simulink model "VehicleModel"  (R2016b)
settings: Solver=FixedStepAuto  StartTime=0.0  StopTime=t_EndSimulation  FixedStep=base_dT  MaxStep=0.01  RelTol=1e-3  EnableMultiTasking=on
values from neighbouring files (symbols this model uses):
  b_E2C_inloop = Simulink.Parameter    [VehicleModelInit.m]
  b_Engine_in_loop = Simulink.Parameter    [VehicleModelInit.m]
  b_initialize_distance_t_startsim = Simulink.Parameter    [VehicleModelInit.m]
  b_Ne_in_loop = Simulink.Parameter    [VehicleModelInit.m]
  b_TTB_in_loop = Simulink.Parameter    [VehicleModelInit.m]
  b_use_acc = Simulink.Parameter    [VehicleModelInit.m]
  b_use_acc_hardset = Simulink.Parameter    [VehicleModelInit.m]
  base_dT = Simulink.Parameter    [VehicleModelInit.m]
  c_acc_d_hdw = Simulink.Parameter    [VehicleModelInit.m]
  c_acc_hdw = Simulink.Parameter    [VehicleModelInit.m]
  c_EngFricCoef = PARS.c_EngFricCoef    [VehicleModelInit.m]
  c_EngFricCoefd = PARS.c_EngFricCoefd    [VehicleModelInit.m]
  d_Ne_max = Simulink.Parameter    [VehicleModelInit.m]
  d_Ne_min = Simulink.Parameter    [VehicleModelInit.m]
  Driver_TuneG1 = PARS.Driver_TuneG1    [VehicleModelInit.m]
  Driver_TuneG2 = PARS.Driver_TuneG2    [VehicleModelInit.m]
  Driver_TuneG3 = PARS.Driver_TuneG3    [VehicleModelInit.m]
  Driver_TuneG_aw = PARS.Driver_TuneG_aw    [VehicleModelInit.m]
  E2C_c2_dTB = Simulink.Parameter    [VehicleModelInit.m]
  E2C_c_dTB = Simulink.Parameter    [VehicleModelInit.m]
  E2C_CycleTimespan = Simulink.Parameter    [VehicleModelInit.m]
  E2C_initializeRelDist = Simulink.Parameter    [VehicleModelInit.m]
  E2C_SpeedShape = Simulink.Parameter    [VehicleModelInit.m]
  E2C_Trap_CycleAcceEndAlpha = Simulink.Parameter    [VehicleModelInit.m]
  E2C_Trap_CycleAcceStartAlpha = Simulink.Parameter    [VehicleModelInit.m]
  E2C_Trap_CycleDeceEndAlpha = Simulink.Parameter    [VehicleModelInit.m]
  E2C_Trap_CycleDeceStartAlpha = Simulink.Parameter    [VehicleModelInit.m]
  E2C_V_High_kmh = Simulink.Parameter    [VehicleModelInit.m]
  E2C_V_Low_kmh = Simulink.Parameter    [VehicleModelInit.m]
  E2C_V_max = Simulink.Parameter    [VehicleModelInit.m]
  E2C_V_min = Simulink.Parameter    [VehicleModelInit.m]
  FTP_speed_1sec = [FTP_speed_once.speed;Idle_speed_once;FTP_speed_once.speed;Idle_speed_once;FTP_speed_once.speed]    [VehicleModelInit.m]
  mass = 3123*1.3    (= 4059.9)    [VehicleModelInit.m]
  T_ACC_TuneG1_data = Simulink.Parameter    [VehicleModelInit.m]
  T_ACC_TuneG1_pt = Simulink.Parameter    [VehicleModelInit.m]
  T_ACC_TuneG2_data = Simulink.Parameter    [VehicleModelInit.m]
  T_ACC_TuneG2_pt = Simulink.Parameter    [VehicleModelInit.m]
  t_StartSimulation = Simulink.Parameter    [VehicleModelInit.m]
  T_TB_ego_ini = Simulink.Parameter    [VehicleModelInit.m]
  T_TB_OffSet = Simulink.Parameter    [VehicleModelInit.m]
  tau_EngTorque = Simulink.Parameter    [VehicleModelInit.m]
  tau_Ne = Simulink.Parameter    [VehicleModelInit.m]
  tau_pedal_dem = Simulink.Parameter    [VehicleModelInit.m]
  VESP_MD = x0.VESP    [VehicleModelInit.m]
undefined symbols (not defined in the file or in its folder): Continuous, DiscIntNeverNeededParam, initializeRelDist, p_ego_ini, p_lead_ini, PedalMapMD, r_w, Simulation_dT, spsSampleAndHoldModel, v_lead_ini, x0
libraries: simulink x9, spsEdgeDetectorModel x6, dspsigops x1
(part 1 of 7)
settings Model: Creator=akshart  LastModifiedBy=Hcn
settings DataIOCC: LimitDataPoints=on  SaveFormat=Array  SignalLoggingSaveFormat=ModelDataLogs
settings OptimizationCC: ExpressionDepthLimit=2147483647  InitFltsAndDblsToZero=on  LifeSpan=inf
settings DebuggingCC: UnderspecifiedInitializationDetection=Classic  MergeDetectMultiDrivingBlocksExec=none  SolverPrmCheckMsg=warning  FcnCallInpInsideContextMsg=warning  StateNameClashWarn=warning  SFUnexpectedBacktrackingDiag=warning  SFNoUnconditionalDefaultTransitionDiag=warning  SFExecutionAtInitializationDiag=none
settings HardwareCC: ProdBitPerPointer=32  ProdBitPerSizeT=32  ProdBitPerPtrDiffT=32  ProdLargestAtomicFloat=None  ProdIntDivRoundTo=Undefined  ProdEndianess=Unspecified  ProdWordSize=32  ProdHWDeviceType=32-bit Generic
settings ModelReferenceCC: PropagateSignalLabelsOutOfModel=off
settings GRTTargetCC: TargetLangStandard=C89/C90 (ANSI)  GeneratePreprocessorConditionals=Disable all  CombineOutputUpdateFcns=off  GRTInterface=on
settings ConfigComp: CovMetricSettings=dw  CovHtmlReporting=on  CovSaveCumulativeToWorkspaceVar=on  CovSaveSingleToWorkspaceVar=on  CovExternalEMLEnable=off  CovSFcnEnable=off

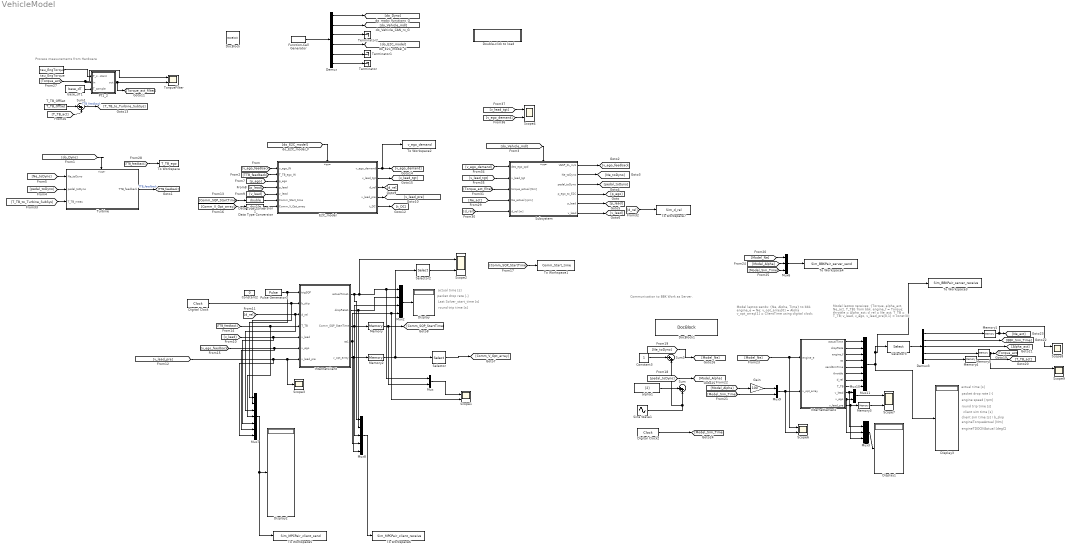
== system VehicleModel ==
  note: Process measurements from Hardware
  note: actual time [s]
  note: packet drop rate [-]
  note: Last Solver_start_time [s]
  note: round trip time [s]
  note: Communication to BBK
      | Work as Server.
  note: Model laptop sends:
      | {Ne, Alpha, Time} to bbk.
      | engine_e = Ne;
      | v_opt_array[0] = Alpha
      | v_opt_array[1] = ClientTime using digital clock;
  note: packet drop rate [-]
  note: actual time [s]
  note: engine speed [rpm]
  note: round trip time [s]
  note: client sim time [s] / b_skip
  note: engineTorqueActual [Nm]
  note: Model laptop receives:
      | {Torque, alpha_act, Ne_act, T_TB} from bbk.
      | engine_f = Torque;
      | throttle = Alpha_act;
      | d_rel = Ne_act;
      | T_TB = T_TB;
      | v_lead, v_ego, v_lead_pre[0,1] = const(0);
  note: engineTDOCINActual [degC]
  note: client sim time [s]
  Constant2 : Constant  Value=0
  Constant3 : Constant
  Data Type Conversion : DataTypeConversion  OutDataTypeStr=double
  Data Type Conversion1 : DataTypeConversion  OutDataTypeStr=double
  Demux : Demux  Outputs=6
  Demux3 : Demux  Outputs=5
  Digital Clock : DigitalClock  SampleTime=base_dT
  Digital Clock2 : DigitalClock  SampleTime=base_dT
  Display{,1..3} (4 alike) : Display
  DocBlock : simulink/Model-Wide Utilities/DocBlock  DocumentType=Text
      content=|
      | Type your documentation here
      |
      | Time                Version Note
      | 101019T1524         Change Ne profile to be slower by changing Driver_Rsl.
      | 101519T2324         Change torque converter torque_ratio in deceleration to make decel Ne fit better.
      | 102219T1600         Integrate solver in Intern_v11 with follower model.
      | 102419T1340         Replace the follower model with 102219T1630 follower model.
      |                     change "off-delay" block to make it run-able in function-call-subsys.
      |                     change multiple continuous solver/integrator to discrete time.
      |                     change multiple delay to discrete time.
      |                     solve "computation loop" problem.
      |                     remove global data store "solver_exec_ctr".
      | 102519T1650         Change the P and I gain for driver_model to be doubled.
      |                     And then changed back, because with the old P and I gains, fuel matches better with data.
      |                     To solve the Ne and speed tracking problem, saturate Ne integrator by 600 and 3400.
      | 102819T1200         Ddd saturation to match idle fuel, only affect fuel consumption number, do not affect driveline.
      |                     Change GearShifting model to have upshift limits: 1600,1800rpm.
      |                     Second bag when vehicle at move (MD.VESP_mph/2.236>=1.5m/s) fuel consumption:
      |                     data fuel at move is -- 764.1621 [g]
      |                     simulink fuel at move is -- 776.5815 [g], +1.63% error.
      | 102819T2340         Change the "follow vehicle1"-->"gain"0.44 place to before acce_filter.
      |                     Previously "filtered_acce" has unit mph/s...
      |                     Change "follow vehicle1"-->"time constant" from 0.5s to 2s.
      |                     data fuel at move is -- 764.5319 [g]
      |                     simulink fuel at move is -- 771.5589 [g], +1.0% error.
      | 102919T1500         -Add substraction for E2C_tiSolverPeriod_C. Because stateflow will add 1 base_dT step.
      |                     Use SendDemand on "E2C_model" subsys to avoid delay introduced by solver_end_time.
      |                     Add function-call subsystem in "E2C_model/solver".
      |                     This way will syncronize with v_ego_array output, and
      |                     update once new optimal v_ego_array is available.
      |                     -"E2C_model/solver/Send  V_demand", add "Matlab Function1" to
      |                     use previous optimal speed as current target speed.
      | 102919T1700         -In previous version, used delayed(v_opt)(1) as previous optimal speed.
      |                     But should be using v_opt(solver_start-delayed(solver_start) ).
      |                     Modified in this version.
      |                     Note: based on solver_start_time to update v_opt_array.
      |                     If solver starts base_dT(s) after solver ends, then correct.
      | 102919T2100         -In previous version, used delayed(v_opt)(1) as previous optimal speed.
      |                     But should be using v_opt(solver_start-delayed(solver_start) ).
      |                     -Use solver_end_time to update v_opt_array.
      | 103119T1400         -Moved leader system out of E2C
      |                     Put leader subsys and Follower subsystem into one function-call system.
      |                     -Compared results from mpcqpsolver and quadprog, final traces are extremely similar. see
      |                     PlatoonModel_Chunan_2016b_102919Txxxx_19_10_31_14_48,PlatoonModel_Chunan_2016b_102919Txxxx_19_10_31_16_22.
      |                     mpcqpsolver is much faster than quadprog.
      | 110519T1100         -in E2C_model, add option for using triditional ACC.
      |                     Add vars b_use_acc,c_acc_hdw.
      |                     changed .m file for setting parameters.
      | 111119T1200         -in E2C_model, add condition for if t_>t_startsimulation.
      |                     only start after 498s.
      |                     -In subsys, change Driver_TuneG1,Driver_TuneG2 to be calibration vars.
      |                     -make V_Opt_Array_modify to be base_dT_delayed(previous V_Opt_Array_modify). Avoid jumps when v_opt updates.
      |                     -PARS.Driver_TuneG1 = 0.015*16;PARS.Driver_TuneG2 = 5;
      |                     with w=0, much smoother optimal speed than before.
      | 111919T1000         -Dyno subsystem change maps for calculating T_TB.
      | 112119T1155         -Add "ToWorkspace" nodes for TTBego, and solver outputs.
      | Client_112619T1415  -Created from PlatoonModel_Chunan_2016b_112119T1155 and InternetClient_112619T1300.
      |                     -Contains the whole vehicle model.
      |                     -Set up memory for CommOut_V_Opt_Array to align change for CommOut_V_Opt_Array and Comm_Start_Time.
      | Solver_112619T1415  -Created.
      |                     -Add semicolon in state flow to avoid printing intermediate variables.
      | C/S_122019T1424     -Add to resolve rtt issue. Not very useful on full model.:
      |                             while (myIns.simTime > timeNow*1)
      |                          {
      |                              QueryPerformanceCounter(&LItNow);
      |                              timeNow = ((double)(LItNow.QuadPart - G.LIstartTime.QuadPart)) / ((double)(G.LIticksPerSecond.QuadPart)) ;
      |                          }
      | %%%%%%%%%%%%%%%%%%%%%%%%%%%%%%%%%%%%%%%%%%%%%%%%%%%%%%%%%%%%%%%%%%%%%%%%%%
      | %                        3-computer setup                                %
      | %%%%%%%%%%%%%%%%%%%%%%%%%%%%%%%%%%%%%%%%%%%%%%%%%%%%%%%%%%%%%%%%%%%%%%%%%%
      | Model_01022020T1343
      |                     -Add Solver block (to bbk).
  DocBlock1 : simulink/Model-Wide Utilities/DocBlock  DocumentType=Text
      content=|
      | 110719T1200         -Finish chart for customized process control
      | 110719T1500         -use Ts=0.1(hardcoded), run server model alone, process control works with EgoFol=1.
      | 110719T1630         -use Ts=base_dT=0.01, run server & client. EgoFol=1.
      | 111119T1200         -Use last_v_opt(solver_start-delayed(solver_start) ) as current v_ego_tgt.
      |                     -Put the modification in Send V_demand subsys.
      |                     -Avoid using another block with detectchange in solver_end_time to trigger this modification.
      |                     -Clean the model and setup communication input/output ports (magenta)
      |                     -Modify Solver_Control so that EgoFol=0 case also works
      | 111119T2200         -Comment out "simulink execution control"
      |                     -If at one step "solver_exec_time>1s", the delay will cumulate
      |                     -need logic control in client to decide whether to skip a trigger.
      | 111219T1300         -Use Client time to set b_termQP.
      |                     -Set E2C_DeltaT=0.3s, save 0.3s for communication
      |                     -Cannot reset if one communication takes long time.
      | Client_112619T1415  -Created from PlatoonModel_Chunan_2016b_112119T1155 and InternetClient_112619T1300.
      |                     -Contains the whole vehicle model.
      |                     -Set up memory for CommOut_V_Opt_Array to align change for CommOut_V_Opt_Array and Comm_Start_Time.
      | Solver_112619T1415  -Created.
      |                     -Add semicolon in state flow to avoid printing intermediate variables.
      | Solver_112719T1142  -Add solver_ctr to workspace
      |                     -Do 10 "dosolver" in 1 step to compensate for base_dT=0.1s. If base_dT=0.01, use 1 dosolver.
      | Solver_112719T2200  -PlatoonModel_Chunan_2016b_112719T2200_solver/Send  V_demand/Triggered Subsystem.
      |                     Change also ceil(current_time-last_start_time).
      | C/S_122019T1424     -Add to resolve rtt issue. Not very useful on full model.:
      |                             while (myIns.simTime > timeNow*1)
      |                          {
      |                              QueryPerformanceCounter(&LItNow);
      |                              timeNow = ((double)(LItNow.QuadPart - G.LIstartTime.QuadPart)) / ((double)(G.LIticksPerSecond.QuadPart)) ;
      |                          }
      | C+S_122019T1618     -Put original solver and client into one system.
      |                     -Now the sent information are place holders to maintain dimension.
      |                     -Finally if this works, the client will be BBK and only sends
      |                     torque, TTB. Solver sends Ne, Alpha.
      | S_122819T1229 (C_122019T1618)
      |                     -Apply changes from Tulga in email "reducing delay further" to 122019T1618.
      |                     -rrt maintains to be 0.02s = base_dT.
      | S_122819T1301 (C_122019T1424)
      |                     -Apply changes from Tulga in email "reducing delay further" to 122019T1424.
      |                     -rrt drops to 0.02s = base_dT.
      |                     -But optimization result is still bad.
      |                     Does not recover optimal results similar to platoonmodel(without interenet),
      |                     like in version S_122819T1229.
      |                     -(!!!)switch Commin_v_lead and v_ego_highfreq at output of InternetServer1 demux.
      | %%%%%%%%%%%%%%%%%%%%%%%%%%%%%%%%%%%%%%%%%%%%%%%%%%%%%%%%%%%%%%%%%%%%%%%%%%
      | %                        3-computer setup                                %
      | %%%%%%%%%%%%%%%%%%%%%%%%%%%%%%%%%%%%%%%%%%%%%%%%%%%%%%%%%%%%%%%%%%%%%%%%%%
  Double-click to load : Subsystem
      settings: OpenFcn=if exist('vesim_init')==2,vesim_init;end;
      mask Help: This block runs/ndes_init.m file in the main directory
      mask Display: disp('Load Input Data')
  E2C_model : Subsystem
  Function-Call Generator : simulink/Ports & Subsystems/Function-Call Generator  sample_time=-1  numberOfIterations=1
  Gain : Gain  Gain=100
  InternetClient : Subsystem  mask(20-sim 4.6 S-Function block){}
      mask help:
      | This block is generated by the 20-sim Matlab Code Generator.
      |
      | * look under the mask to get information on the ports
      | * press Help for more detailed information
      | * the parameters of this block are:
      mask Help:
      | This block is generated by the 20-sim Matlab Code Generator<br>
      | The block parameters are:<br><blockquote></blockquote>
      | Generated at:<br>
      | <blockquote><b>date:  </b>June 14, 2017<br>
      | <b>time:  </b>4:16:43 PM<br></blockquote>
      | From the following 20-sim model:<br>
      | <blockquote><b>submodel:  </b>InternetServer<br>
      | <b>model:  </b>export to Simulink - UM<br>
      | <b>file:  </b>C:\Users\Tulga Ersal\Desktop\For Xueru\export to Simulink - UM.emx<br>
      | <b>experiment:  </b>C:\Users\Tulga Ersal\Desktop\For Xueru\export to Simulink - UM.emx<br></blockquote>
      | Using the following 20-sim license:<br>
      | <blockquote><b>user:  </b>The University of Michigan<br>
      | <b>from:  </b>20-sim 4.6 Student License<br>
      | <b>build: </b>4.6.1.6898<br></blockquote>
  InternetServer2 : Subsystem  mask(20-sim 4.6 S-Function block){}
      mask help:
      | This block is generated by the 20-sim Matlab Code Generator.
      |
      | * look under the mask to get information on the ports
      | * press Help for more detailed information
      | * the parameters of this block are:
      mask Help:
      | This block is generated by the 20-sim Matlab Code Generator<br>
      | The block parameters are:<br><blockquote></blockquote>
      | Generated at:<br>
      | <blockquote><b>date:  </b>June 14, 2017<br>
      | <b>time:  </b>4:16:43 PM<br></blockquote>
      | From the following 20-sim model:<br>
      | <blockquote><b>submodel:  </b>InternetServer<br>
      | <b>model:  </b>export to Simulink - UM<br>
      | <b>file:  </b>C:\Users\Tulga Ersal\Desktop\For Xueru\export to Simulink - UM.emx<br>
      | <b>experiment:  </b>C:\Users\Tulga Ersal\Desktop\For Xueru\export to Simulink - UM.emx<br></blockquote>
      | Using the following 20-sim license:<br>
      | <blockquote><b>user:  </b>The University of Michigan<br>
      | <b>from:  </b>20-sim 4.6 Student License<br>
      | <b>build: </b>4.6.1.6898<br></blockquote>
  Memory : Memory  InheritSampleTime=on  LinearizeAsDelay=on
  Memory1 : Memory  X0=600
  Memory2 : Memory  X0=zeros(40,1)  InheritSampleTime=on  LinearizeAsDelay=on
  Memory3 : Memory  X0=zeros(2,1)  InheritSampleTime=on  LinearizeAsDelay=on
  Memory4 : Memory  X0=200  InheritSampleTime=on  LinearizeAsDelay=on
  Memory5 : Memory  InheritSampleTime=on  LinearizeAsDelay=on
  Mux : Mux  Inputs=2
  Mux10 : Mux  Inputs=2
  Mux11 : Mux  Inputs=8
  Mux2 : Mux
  Mux3 : Mux  Inputs=3
  Mux6 : Mux  Inputs=3
  Mux7 : Mux  Inputs=7
  Mux8 : Mux  Inputs=5
  Mux9 : Mux  Inputs=2
  PT1_2 : Subsystem  mask(PT1_1){}
  Pulse Generator1 : DiscretePulseGenerator  PulseType=Time based  Period=1  PulseWidth=20  SampleTime=base_dT
  Scope{1..2,4,6..9} (7 alike) : Scope  NumInputPorts=2
  Scope3 : Scope
  Selector : Selector  InputPortWidth=40  IndexOptions=Index vector (dialog)  Indices=[1:40]  OutputSizes=1
  Selector2 : Selector  InputPortWidth=40  IndexOptions=Index vector (dialog)  Indices=[1:10]  OutputSizes=1
  Selector3 : Selector  InputPortWidth=8  IndexOptions=Index vector (dialog)  Indices=[3,5,6,7,8]  OutputSizes=1
  Sine Wave1 : Sin  SampleTime=0
  Subsystem : Subsystem
  Sum : Sum  Inputs=|++
  Sum1 : Sum  Inputs=|++
  Sum3 : Sum  Inputs=|++
  T_TB_OffSet : Constant  Value=T_TB_OffSet
  Terminator : Terminator
  Terminator1 : Terminator
  Terminator2 : Terminator
  To Workspace : ToWorkspace  VariableName=T_TB_ego  SaveFormat=Structure With Time  SampleTime=-1
  To Workspace1 : ToWorkspace  VariableName=Comm_Start_time  SaveFormat=Structure With Time  SampleTime=-1
  To Workspace2 : ToWorkspace  VariableName=v_ego_demand  SaveFormat=Structure With Time  SampleTime=-1
  To Workspace3 : ToWorkspace  VariableName=Sim_BBKPair_server_receive  SaveFormat=Structure With Time  SampleTime=-1
  To Workspace4 : ToWorkspace  VariableName=Sim_BBKPair_server_send  SaveFormat=Structure With Time  SampleTime=-1
  To Workspace5 : ToWorkspace  VariableName=Sim_MPCPair_client_send  SaveFormat=Structure With Time  SampleTime=-1
  To Workspace6 : ToWorkspace  VariableName=Sim_MPCPair_client_receive  SaveFormat=Structure With Time  SampleTime=-1
  To Workspace7 : ToWorkspace  VariableName=Sim_d_rel  SaveFormat=Structure With Time  SampleTime=-1
  "TorqueFilter " : Scope  NumInputPorts=2
  Turbine : Subsystem  TreatAsAtomicUnit=on
  alpha1 : Constant  Value=[2]  VectorParams1D=off  SampleTime=base_dT
  base_dT1 : Constant  Value=base_dT
  tau_EngTorque : Constant  Value=tau_EngTorque
  wires:
  [v_ego_feedback] -> E2C_model/1(v_ego_IN)
  [TTB_feedback] -> E2C_model/2(T_TB_ego_IN)
  Function-Call Generator/1 -> Demux/1
  Demux/1 -> [do_Dyno]
  Demux/2 -> [do_Vehicle_mdl]
  Demux/3 -> Terminator2/1
  Demux/4 -> [do_E2C_model]
  Demux/5 -> Terminator1/1
  Demux/6 -> Terminator/1
  [Ne_toDyno] -> Turbine/1(Ne_toDyno)
  [pedal_toDyno] -> Turbine/2(pedal_toDyno)
  [do_E2C_model] -> E2C_model/Trigger
  [do_Dyno] -> Turbine/Trigger
  [do_Vehicle_mdl] -> Subsystem/Trigger
  E2C_model/1(v_ego_demand) -> [v_ego_demand], To Workspace2/1
  Subsystem/1(VESP_FL_m/s) -> [v_ego_feedback]
  Subsystem/2(Ne_toDyno) -> [Ne_toDyno]
  Subsystem/3(pedal_toDyno) -> [pedal_toDyno]
  Subsystem/4(p_ego_to_E2C) -> [p_ego]
  [v_lead_tgt] -> Subsystem/2(v_lead_tgt)
  [p_ego] -> E2C_model/3(p_ego)
  Subsystem/5(p_lead) -> [p_lead]
  [p_lead] -> E2C_model/4(p_lead)
  Subsystem/6(v_lead) -> [v_lead]
  [v_lead] -> E2C_model/5(v_lead)
  [v_ego_feedback] -> Mux7/6, InternetClient/6(v_ego)
  [TTB_feedback] -> Mux7/4, InternetClient/4(T_TB)
  [d_rel] -> Mux7/3, InternetClient/3(d_rel)
  InternetClient/3(Comm_SQP_StartTime) -> Mux8/3, Mux2/3, Memory/1
  Memory/1 -> Mux/2, [Comm_SQP_StartTime]
  InternetClient/5(v_opt_array) -> Mux8/5, Memory2/1
  [v_lead] -> Mux7/5, InternetClient/5(v_lead)
  Pulse Generator1/1 -> Mux7/1, InternetClient/1(trigSQP)
  InternetClient/1(actualTime1) -> Mux8/1, Scope2/1, Mux/1, Mux2/1
  InternetClient/2(dropRate1) -> Mux8/2, Mux2/2
  InternetClient/4(rtt1) -> Scope1/2, Mux2/4, Mux8/4
  Mux2/1 -> Display/1
  E2C_model/3(d_rel) -> [d_rel]
  E2C_model/4(v_lead_pre) -> [v_lead_pre]
  [Comm_SQP_StartTime] -> Data Type Conversion1/1
  [Comm_V_Opt_array] -> Data Type Conversion/1
  Data Type Conversion/1 -> E2C_model/7(Comm_V_Opt_array)
  Data Type Conversion1/1 -> E2C_model/6(Comm_Start_time)
  Memory2/1 -> Selector/1, Selector2/1
  Mux/1 -> Scope1/1
  [Comm_SQP_StartTime] -> To Workspace1/1
  Selector/1 -> [Comm_V_Opt_array]
  Selector2/1 -> Scope2/2
  Digital Clock/1 -> Mux7/2, InternetClient/2(b_skip)
  Mux6/1 -> To Workspace4/1
  Mux7/1 -> Display2/1, To Workspace5/1
  Mux8/1 -> To Workspace6/1
  Demux3/1 -> Memory1/1
  Demux3/2 -> [BBK_Sim_Time]
  Demux3/3 -> [Alpha_act]
  InternetServer2/3(engine_f) -> Mux11/3
  InternetServer2/4(rtt) -> Mux11/4
  InternetServer2/2(dropRate) -> Mux11/2
  InternetServer2/5(sendSimTime) -> Mux11/5
  InternetServer2/1(actualTime) -> Mux11/1
  InternetServer2/6(throttle) -> Mux11/6
  Mux11/1 -> Display3/1, To Workspace3/1, Selector3/1
  InternetServer2/7(d_rel) -> Mux11/7
  InternetServer2/8(T_TB) -> Mux11/8
  InternetServer2/9(v_lead) -> Mux3/1, Mux10/1
  InternetServer2/10(v_ego) -> Mux3/2, Mux10/2
  InternetServer2/11(v_lead_pre) -> Mux3/3, Memory3/1
  alpha1/1 -> Sum/1
  [Model_Ne] -> Scope6/1, InternetServer2/1(engine_e)
  Selector3/1 -> Demux3/1
  Demux3/5 -> Memory4/1
  Memory4/1 -> [T_TB_act]
  Mux9/1 -> Scope6/2, InternetServer2/2(v_opt_array)
  Sine Wave1/1 -> Sum3/2, Sum/2
  Memory3/1 -> Scope7/2
  Digital Clock2/1 -> [Model_Sim_Time]
  [Model_Sim_Time] -> Mux9/2
  [pedal_toDyno] -> [Model_Alpha]
  Constant3/1 -> Sum3/1
  [Ne_toDyno] -> [Model_Ne]
  [Model_Ne] -> Mux6/1
  [Model_Alpha] -> Mux6/2
  [Model_Sim_Time] -> Mux6/3
  Mux10/1 -> Scope7/1
  Mux3/1 -> Display1/1
  E2C_model/5(t_DC) -> [t_DC]
  [Model_Alpha] -> Gain/1
  Gain/1 -> Mux9/1
  [TTB_feedback] -> To Workspace/1
  PT1_2/1(out) -> [Torque_act_filter], "TorqueFilter "/2
  Demux3/4 -> Memory5/1
  Memory1/1 -> Scope8/1, [Ne_act]
  Memory5/1 -> Scope9/1, [Torque_act]
  [Torque_act] -> "TorqueFilter "/1, PT1_2/2(in)
  tau_EngTorque/1 -> PT1_2/1(T_constant)
  base_dT1/1 -> PT1_2/3(T_sample)
  [d_rel] -> To Workspace7/1
  [v_lead_pre] -> Mux7/7, Scope3/1, InternetClient/7(v_lead_pre)
  [Ne_act] -> Subsystem/4(Ne_actual [rpm])
  [T_TB_act] -> Sum1/2
  T_TB_OffSet/1 -> Sum1/1
  Sum1/1 -> [T_TB_to_Turbine_SubSys]  "TTB_feedback"
  [d_rel] -> Subsystem/5(d_rel [m])
  [Torque_act_filter] -> Subsystem/3(torque_actual [Nm])
  Turbine/1(TTB_feedback) -> [TTB_feedback]  "TTB_feedback"
  [T_TB_to_Turbine_SubSys] -> Turbine/3(T_TB_meas)
  [v_ego_demand] -> Subsystem/1(des_ego_spd)
  E2C_model/2(v_lead_tgt) -> [v_lead_tgt]
  [v_lead_tgt] -> Scope4/1
  [v_ego_demand] -> Scope4/2

== system VehicleModel/Double-click to load ==
  note: double_click to load

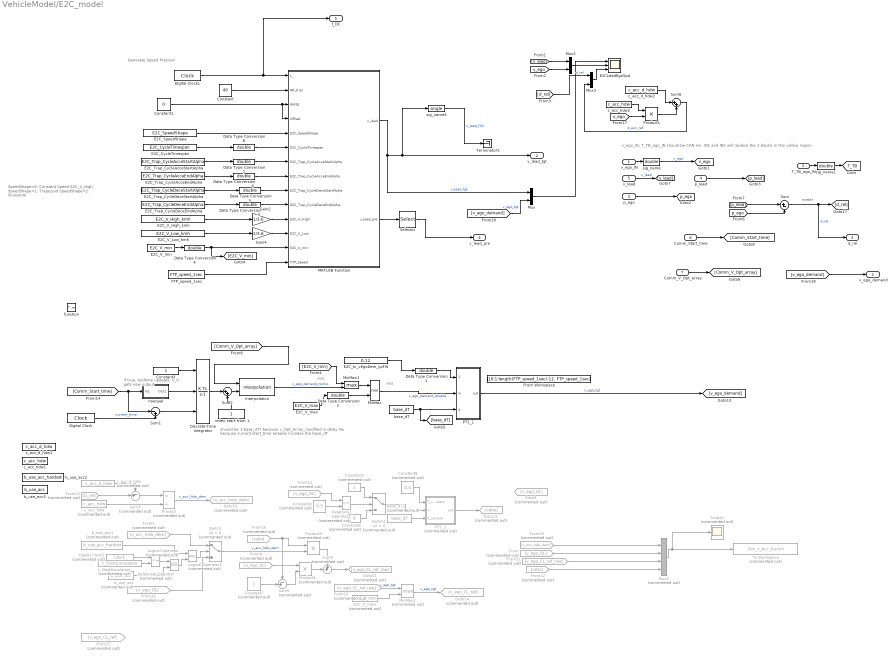
== system VehicleModel/E2C_model ==
  note: should be 1-base_dT? because v_Opt_Array_modified is delay
      | No because current-start_time already includes the base_dT
  note: if true, endtime updates,
      | v_0 gets new output
  note: SpeedShape=0: Constant Speed E2C_V_High
      | SpeedShape=1: Trapezoid
      | SpeedShape=2: Sinusoide
  note: meter
  note: Generate Speed Preview
  note: v_ego_IN, T_TB_ego_IN should be CAN ms. IN1 and IN2 will replace the 2 blocks in this
      | yellow region.
  note: m/s
  note: m/s
  v_ego_IN : Inport
  T_TB_ego_IN : Inport  Port=2
  p_ego : Inport  Port=3
  p_lead : Inport  Port=4
  v_lead : Inport  Port=5
  Comm_Start_time : Inport  Port=6
  Comm_V_Opt_array : Inport  Port=7
  function : TriggerPort  TriggerType=function-call  VariantControl=Variant
  Constant : Constant  Value=40
  Constant1 : Constant  Value=0
  Constant3 : Constant  OutDataTypeStr=double
  Constant4 : Constant  Commented=on  Value=0.5
  Constant5 : Constant  Commented=on
  Constant6 : Constant  Commented=on  Value=0
  Constant7 : Constant  Commented=on
  Constant8 : Constant  Commented=on  Value=0.4
  Data Type Conversion{1..8} (8 alike) : DataTypeConversion  OutDataTypeStr=double
  Digital Clock : DigitalClock  SampleTime=-1
  Digital Clock1 : DigitalClock  SampleTime=-1
  Digital Clock2 : DigitalClock  Commented=on  SampleTime=-1
  Discrete-Time Integrator : DiscreteIntegrator  ExternalReset=rising  InitialConditionSource=external  SampleTime=-1  ICPrevOutput=DiscIntNeverNeededParam  ICPrevScaledInput=DiscIntNeverNeededParam
  E2CLeadEgoSpd : Scope  NumInputPorts=3
  E2C_CycleTimespan : Constant  Value=E2C_CycleTimespan  OutDataTypeStr=single
  E2C_SpeedShape : Constant  Value=E2C_SpeedShape  OutDataTypeStr=uint8
  E2C_Trap_CycleAcceEndAlpha : Constant  Value=E2C_Trap_CycleAcceEndAlpha  OutDataTypeStr=single
  E2C_Trap_CycleAcceStartAlpha : Constant  Value=E2C_Trap_CycleAcceStartAlpha  OutDataTypeStr=single
  E2C_Trap_CycleDeceEndAlpha : Constant  Value=E2C_Trap_CycleDeceEndAlpha  OutDataTypeStr=single
  E2C_Trap_CycleDeceStartAlpha : Constant  Value=E2C_Trap_CycleDeceStartAlpha  OutDataTypeStr=single
  E2C_V_High_kmh : Constant  Value=E2C_V_High_kmh  OutDataTypeStr=single
  E2C_V_Low_kmh : Constant  Value=E2C_V_Low_kmh  OutDataTypeStr=single
  E2C_V_max : Constant  Value=E2C_V_max  OutDataTypeStr=double
  E2C_V_min : Constant  Value=E2C_V_min  OutDataTypeStr=single
  E2C_V_min2 : Constant  Commented=on  Value=E2C_V_min
  E2C_tc_vEgoDem_LpFilt : Constant  Value=0.12  OutDataTypeStr=single
  FTP_speed_1sec : Constant  Value=FTP_speed_1sec
  From{,9,11,16} (4 alike) : From  Commented=on  GotoTag=v_ego_OL
  From Workspace : FromWorkspace  VariableName=[[0:1:length(FTP_speed_1sec)-1]', FTP_speed_1sec]
  From10 : From  Commented=on  GotoTag=v_acc_hdw_dem
  From12 : From  Commented=on  GotoTag=d_rel
  From13 : From  Commented=on  GotoTag=v_ego_CL_ref_raw
  From15 : From  Commented=on  GotoTag=ratio
  From21 : From  Commented=on  GotoTag=v_ego_CL_ref_raw
  From22 : From  Commented=on  GotoTag=ratio
  From25 : From  Commented=on  GotoTag=v_ego_CL_ref
  From5 : From  Commented=on  GotoTag=v_acc_hdw_dem
  Gain2 : Gain  Gain=1/3.6  OutDataTypeStr=double
  Gain4 : Gain  Gain=1/3.6  OutDataTypeStr=double
  Goto10 : Goto  Commented=on  GotoTag=v_acc_hdw_dem
  Goto11 : Goto  Commented=on  GotoTag=v_ego_CL_ref_raw
  Goto12 : Goto  Commented=on  GotoTag=ratio
  Goto14 : Goto  Commented=on  GotoTag=v_ego_CL_ref
  Goto9 : Goto  Commented=on  GotoTag=v_ego_OL
  Interpolation : dspsigops/Interpolation  InterpSource=Input port  InterpPoints=[1.1 4.8 2.67 1.6 3.2]'  InterpMode=Linear  InterpL=3  InterpR=3  InterpAlpha=0.5  InvalidMode=Clip
  Logical Operator : Logic  Commented=on  Operator=OR  AllPortsSameDT=off  OutDataTypeStr=boolean
  Logical Operator1 : Logic  Commented=on  AllPortsSameDT=off  OutDataTypeStr=boolean
  MATLAB Function : MATLAB Function  TreatAsAtomicUnit=on
  MinMax : MinMax  Inputs=2
  MinMax1 : MinMax  Function=max  Inputs=2
  MinMax2 : MinMax  Commented=on  Function=max  Inputs=2
  Mux : Mux  Inputs=2
  Mux1 : Mux  Commented=on
  Mux2 : Mux  Inputs=2
  Mux3 : Mux  Inputs=2
  PT1_1 : Subsystem  mask(PT1_1){}
  PT1_2 : Subsystem  Commented=on  mask(PT1_1){}
  Product : Product  Commented=on  Inputs=*/
  Product1 : Product
  Product3 : Product  Commented=on
  Product4 : Product  Commented=on
  Relational Operator : RelationalOperator  Commented=on  Operator=<=  OutDataTypeStr=boolean  RndMeth=Simplest
  Relational Operator1 : RelationalOperator  Commented=on  OutDataTypeStr=boolean  RndMeth=Simplest
  Scope1 : Scope  Commented=on
  Selector : Selector  InputPortWidth=41  IndexOptions=Index vector (dialog)  Indices=[1:40]  OutputSizes=1
  Sum : Sum  Inputs=|+-
  Sum1 : Sum  Inputs=|-+  OutDataTypeStr=double
  Sum2 : Sum  Inputs=|++
  Sum3 : Sum  Commented=on  Inputs=-+|
  Sum4 : Sum  Commented=on  Inputs=++|
  Sum5 : Sum  Commented=on  Inputs=-+|
  Sum6 : Sum  Inputs=|++
  Switch : Switch  Commented=on  Criteria=u2 > Threshold
  Switch1 : Switch  Commented=on  Criteria=u2 > Threshold
  Terminator5 : Terminator
  To Workspace : ToWorkspace  Commented=on  VariableName=Sim_v_Acc_bunch  SaveFormat=Structure With Time  SampleTime=-1
  b_use_acc : Constant  Commented=on  Value=b_use_acc
  b_use_acc1 : Constant  Commented=on  Value=b_use_acc_hardset
  b_use_acc2 : Constant  Value=b_use_acc_hardset
  b_use_acc3 : Constant  Value=b_use_acc
  base_dT : Constant  Value=base_dT
  base_dT1 : Constant  Commented=on  Value=base_dT
  c_acc_d_hdw : Constant  Commented=on  Value=c_acc_d_hdw
  c_acc_d_hdw1 : Constant  Value=c_acc_d_hdw
  c_acc_d_hdw2 : Constant  Value=c_acc_d_hdw
  c_acc_hdw : Constant  Commented=on  Value=c_acc_hdw
  c_acc_hdw1 : Constant  Value=c_acc_hdw
  c_acc_hdw2 : Constant  Value=c_acc_hdw
  index start from 1 : Constant  OutDataTypeStr=double
  noequal : Subsystem
      mask Display: fprintf('U ~= U/z')
  sig_name : DataTypeConversion  OutDataTypeStr=double
  sig_name1 : DataTypeConversion  OutDataTypeStr=double
  sig_name4 : DataTypeConversion  OutDataTypeStr=single
  t_StartSimulation : Constant  Commented=on  Value=t_StartSimulation
  v_ego_demand : Outport
  v_lead_tgt : Outport  Port=2
  d_rel : Outport  Port=3
  v_lead_pre : Outport  Port=4
  t_DC : Outport  Port=5
  tag scope: T_TB=global, p_ego=global, v_ego=global
  wires:
  [p_ego] -> Sum/2
  [p_lead] -> Sum/1
  T_TB_ego_IN/1 -> sig_name1/1
  sig_name1/1 -> [T_TB]
  v_ego_IN/1 -> sig_name/1
  p_ego/1 -> [p_ego]
  Sum/1 -> d_rel/1, [d_rel]  "d_rel"
  Digital Clock/1 -> Sum1/2  "current_time"
  Constant/1 -> MATLAB Function/2(NP_trial)
  Constant1/1 -> MATLAB Function/4(Offset), MATLAB Function/3(RMSE)
  E2C_SpeedShape/1 -> MATLAB Function/5(E2C_SpeedShape)
  E2C_CycleTimespan/1 -> Data Type Conversion8/1
  E2C_Trap_CycleAcceStartAlpha/1 -> Data Type Conversion7/1
  E2C_Trap_CycleAcceEndAlpha/1 -> Data Type Conversion6/1
  E2C_Trap_CycleDeceStartAlpha/1 -> Data Type Conversion5/1
  E2C_Trap_CycleDeceEndAlpha/1 -> Data Type Conversion3/1
  E2C_V_Low_kmh/1 -> Gain4/1
  E2C_V_min/1 -> Data Type Conversion4/1
  Data Type Conversion4/1 -> [E2C_V_min], MATLAB Function/13(E2C_V_min)
  Gain2/1 -> MATLAB Function/11(E2C_V_High)
  Gain4/1 -> MATLAB Function/12(E2C_V_Low)
  MATLAB Function/2(v_lead_pre) -> Selector/1
  MATLAB Function/1(v_lead) -> Mux/1, v_lead_tgt/1, sig_name4/1  "v_lead_tgt"
  FTP_speed_1sec/1 -> MATLAB Function/14(FTP_Speed)
  E2C_V_High_kmh/1 -> Gain2/1
  Data Type Conversion3/1 -> MATLAB Function/10(E2C_Trap_CycleDeceEndAlpha)
  Data Type Conversion6/1 -> MATLAB Function/8(E2C_Trap_CycleAcceEndAlpha)
  Data Type Conversion5/1 -> MATLAB Function/9(E2C_Trap_CycleDeceStartAlpha)
  Data Type Conversion7/1 -> MATLAB Function/7(E2C_Trap_CycleAcceStartAlpha)
  Data Type Conversion8/1 -> MATLAB Function/6(E2C_CycleTimespan)
  sig_name4/1 -> Terminator5/1  "v_lead_f32"
  [Comm_Start_time] -> Sum1/1, noequal/1(In1)
  Discrete-Time Integrator/1 -> Sum2/1
  index start from 1/1 -> Sum2/2
  Sum2/1 -> Interpolation/2
  Constant3/1 -> Discrete-Time Integrator/1
  [E2C_V_min] -> MinMax1/1
  Interpolation/1 -> MinMax1/2  "v_ego_demand_noclip"
  MinMax1/1 -> MinMax/1
  MinMax/1 -> PT1_1/2(in)  "v_ego_demand_double"
  E2C_tc_vEgoDem_LpFilt/1 -> Data Type Conversion1/1
  base_dT/1 -> PT1_1/3(T_sample), [base_dT]
  E2C_V_max/1 -> Data Type Conversion2/1
  Data Type Conversion2/1 -> MinMax/2
  sig_name/1 -> [v_ego]  "v_ego"
  Data Type Conversion1/1 -> PT1_1/1(T_constant)
  Sum1/1 -> Discrete-Time Integrator/3
  noequal/1(Out1) -> Discrete-Time Integrator/2
  [Comm_V_Opt_array] -> Interpolation/1
  p_lead/1 -> [p_lead]
  v_lead/1 -> [v_lead]  "v_lead"
  Mux/1 -> E2CLeadEgoSpd/1
  Mux2/1 -> E2CLeadEgoSpd/2
  c_acc_hdw/1 -> Product/2
  PT1_1/1(out) -> [v_ego_demand]  "v_ego_tgt"
  Digital Clock1/1 -> t_DC/1, MATLAB Function/1(t_)
  [v_lead] -> Mux2/1
  [v_ego] -> Mux2/2
  Selector/1 -> v_lead_pre/1
  Comm_V_Opt_array/1 -> [Comm_V_Opt_array]
  Comm_Start_time/1 -> [Comm_Start_time]
  E2C_V_min2/1 -> MinMax2/2
  Sum3/1 -> Product/1
  From13/1 -> MinMax2/1  "v_ego_tgt"
  t_StartSimulation/1 -> Relational Operator/2
  Digital Clock2/1 -> Relational Operator/1
  Relational Operator/1 -> Logical Operator/1
  b_use_acc/1 -> Logical Operator/2
  Logical Operator/1 -> Logical Operator1/2
  From12/1 -> Sum3/2
  From16/1 -> Switch/3
  Product/1 -> Goto10/1  "v_acc_hdw_dem"
  Product3/1 -> Sum4/1
  Product4/1 -> Sum4/2
  From/1 -> Mux1/2
  From10/1 -> Mux1/1
  From11/1 -> Relational Operator1/1
  Sum4/1 -> Goto11/1
  Relational Operator1/1 -> Switch1/2
  Constant4/1 -> Relational Operator1/2
  base_dT1/1 -> PT1_2/3(T_sample)
  Constant5/1 -> Switch1/1
  Constant6/1 -> Switch1/3
  Switch1/1 -> PT1_2/2(in)
  PT1_2/1(out) -> Goto12/1
  From9/1 -> Product4/1
  Sum5/1 -> Product4/2
  Constant7/1 -> Sum5/2
  Constant8/1 -> PT1_2/1(T_constant)
  From15/1 -> Sum5/1, Product3/1
  c_acc_d_hdw/1 -> Sum3/1
  Switch/1 -> Product3/2  "v_acc_hdw_dem"
  From5/1 -> Switch/1
  [v_ego_demand] -> Mux/2  "v_ego_tgt"
  Mux1/1 -> Scope1/1, To Workspace/1
  From21/1 -> Mux1/3
  Logical Operator1/1 -> Switch/2
  b_use_acc1/1 -> Logical Operator1/1
  From22/1 -> Mux1/4
  MinMax2/1 -> Goto14/1  "v_ego_tgt"
  [v_ego_demand] -> v_ego_demand/1
  c_acc_hdw2/1 -> Product1/1
  [v_ego] -> Product1/2
  Product1/1 -> Sum6/2
  c_acc_d_hdw2/1 -> Sum6/1
  [d_rel] -> Mux3/1  "d_rel"
  Mux3/1 -> E2CLeadEgoSpd/3
  Sum6/1 -> Mux3/2  "d_acc_ref"

== system VehicleModel/InternetClient ==
  trigSQP : Inport
  b_skip : Inport  Port=2
  d_rel : Inport  Port=3
  T_TB : Inport  Port=4
  v_lead : Inport  Port=5
  v_ego : Inport  Port=6
  v_lead_pre : Inport  Port=7
  Demux1 : Demux  Outputs=[1 1 1 1 40 ]
  Mux1 : Mux  Inputs=[1 1 1 1 1 1 40 ]
  S-Function1 : S-Function  FunctionName=InternetClient  SFunctionDeploymentMode=off  EnableBusSupport=off
  actualTime1 : Outport
  dropRate1 : Outport  Port=2
  Comm_SQP_StartTime : Outport  Port=3
  rtt1 : Outport  Port=4
  v_opt_array : Outport  Port=5
  wires:
  Demux1/1 -> actualTime1/1
  Demux1/2 -> dropRate1/1
  Demux1/3 -> Comm_SQP_StartTime/1
  Demux1/4 -> rtt1/1
  S-Function1/1 -> Demux1/1
  trigSQP/1 -> Mux1/1
  b_skip/1 -> Mux1/2
  Mux1/1 -> S-Function1/1
  T_TB/1 -> Mux1/4
  d_rel/1 -> Mux1/3
  v_lead/1 -> Mux1/5
  v_ego/1 -> Mux1/6
  v_lead_pre/1 -> Mux1/7
  Demux1/5 -> v_opt_array/1

== system VehicleModel/InternetServer2 ==
  engine_e : Inport
  v_opt_array : Inport  Port=2
  Demux : Demux  Outputs=[1 1 1 1 1 1 1 1 1 1 2]
  Mux : Mux  Inputs=[1 2 ]
  S-Function : S-Function  FunctionName=InternetServer  SFunctionDeploymentMode=off  EnableBusSupport=off
  actualTime : Outport
  dropRate : Outport  Port=2
  engine_f : Outport  Port=3
  rtt : Outport  Port=4
  sendSimTime : Outport  Port=5
  throttle : Outport  Port=6
  d_rel : Outport  Port=7
  T_TB : Outport  Port=8
  v_lead : Outport  Port=9
  v_ego : Outport  Port=10
  v_lead_pre : Outport  Port=11
  wires:
  engine_e/1 -> Mux/1
  Demux/1 -> actualTime/1
  Demux/2 -> dropRate/1
  Demux/3 -> engine_f/1
  Demux/4 -> rtt/1
  Demux/5 -> sendSimTime/1
  Demux/6 -> throttle/1
  Mux/1 -> S-Function/1
  S-Function/1 -> Demux/1
  Demux/7 -> d_rel/1
  Demux/8 -> T_TB/1
  Demux/9 -> v_lead/1
  Demux/10 -> v_ego/1
  Demux/11 -> v_lead_pre/1
  v_opt_array/1 -> Mux/2

== system VehicleModel/PT1_2 ==
  T_constant : Inport
  in : Inport  Port=2
  T_sample : Inport  Port=3
  map_error_1 : Sum  Inputs=+-  SaturateOnIntegerOverflow=on  InputSameDT=on  OutDataTypeStr=Inherit: Same as first input
  map_error_2 : Sum  Inputs=2  SaturateOnIntegerOverflow=on  InputSameDT=on  OutDataTypeStr=Inherit: Same as first input
  product_1 : Product  Inputs=*/  SaturateOnIntegerOverflow=on  InputSameDT=on  OutDataTypeStr=Inherit: Same as first input
  product_2 : Product  Inputs=**  SaturateOnIntegerOverflow=on  InputSameDT=on  OutDataTypeStr=Inherit: Same as first input
  saturation_1 : Saturate  UpperLimit=1  LowerLimit=0
  unit_delay_1 : UnitDelay  SampleTime=-1
  out : Outport
  wires:
  T_constant/1 -> product_1/2
  T_sample/1 -> product_1/1
  in/1 -> map_error_1/1
  map_error_1/1 -> product_2/2
  product_1/1 -> saturation_1/1
  saturation_1/1 -> product_2/1
  unit_delay_1/1 -> map_error_1/2, map_error_2/2
  map_error_2/1 -> out/1, unit_delay_1/1
  product_2/1 -> map_error_2/1

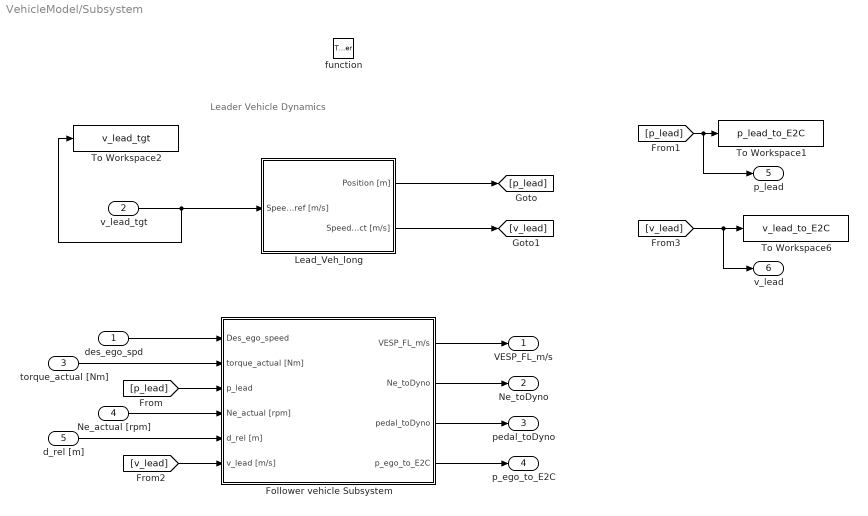
== system VehicleModel/Subsystem ==
  note: Leader Vehicle Dynamics
  des_ego_spd : Inport
  v_lead_tgt : Inport  Port=2
  torque_actual [Nm] : Inport  Port=3
  Ne_actual [rpm] : Inport  Port=4
  d_rel [m] : Inport  Port=5
  function : TriggerPort  TriggerType=function-call  VariantControl=Variant
  Follower vehicle Subsystem : Subsystem  TreatAsAtomicUnit=on
  Lead_Veh_long : Subsystem
  To Workspace1 : ToWorkspace  VariableName=p_lead_to_E2C  SaveFormat=Structure With Time  SampleTime=-1
  To Workspace2 : ToWorkspace  VariableName=v_lead_tgt  SaveFormat=Structure With Time  SampleTime=-1
  To Workspace6 : ToWorkspace  VariableName=v_lead_to_E2C  SaveFormat=Structure With Time  SampleTime=-1
  VESP_FL_m/s : Outport
  Ne_toDyno : Outport  Port=2
  pedal_toDyno : Outport  Port=3
  p_ego_to_E2C : Outport  Port=4
  p_lead : Outport  Port=5
  v_lead : Outport  Port=6
  wires:
  Follower vehicle Subsystem/1(VESP_FL_m/s) -> VESP_FL_m/s/1
  Follower vehicle Subsystem/3(pedal_toDyno) -> pedal_toDyno/1
  Follower vehicle Subsystem/2(Ne_toDyno) -> Ne_toDyno/1
  Lead_Veh_long/1(Position [m]) -> [p_lead]
  v_lead_tgt/1 -> To Workspace2/1, Lead_Veh_long/1(Speed_ref [m/s])
  Follower vehicle Subsystem/4(p_ego_to_E2C) -> p_ego_to_E2C/1
  Lead_Veh_long/2(Speed_act [m/s]) -> [v_lead]
  des_ego_spd/1 -> Follower vehicle Subsystem/1(Des_ego_speed)
  torque_actual [Nm]/1 -> Follower vehicle Subsystem/2(torque_actual [Nm])
  Ne_actual [rpm]/1 -> Follower vehicle Subsystem/4(Ne_actual [rpm])
  d_rel [m]/1 -> Follower vehicle Subsystem/5(d_rel [m])
  [p_lead] -> Follower vehicle Subsystem/3(p_lead)
  [v_lead] -> Follower vehicle Subsystem/6(v_lead [m/s])
  [p_lead] -> p_lead/1, To Workspace1/1
  [v_lead] -> To Workspace6/1, v_lead/1

== system VehicleModel/Turbine ==
  note: Should not use this one for careful simulation tests.
      | This is only needed to setup the code at the first place.
  Ne_toDyno : Inport
  pedal_toDyno : Inport  Port=2
  T_TB_meas : Inport  Port=3
  function : TriggerPort  TriggerType=function-call  VariantControl=Variant
  Constant : Constant  Commented=on  Value=base_dT
  Memory : Memory  Commented=on
  Product : Product  Commented=on  Inputs=/*
  Sum : Sum  Commented=on  Inputs=|-+
  Switch : Switch  Criteria=u2 > Threshold
  TTB : Scope  NumInputPorts=3
  To Workspace8 : ToWorkspace  VariableName=T_TB_ego_Sim  SaveFormat=Structure With Time  SampleTime=-1
  Turbine Thermal : Subsystem  Commented=on
  Turbine Thermal1 : Subsystem
  b_TTB_in_loop : Constant  Value=b_TTB_in_loop  SampleTime=-1
  TTB_feedback : Outport  InitialOutput=200
  wires:
  Turbine Thermal/1(T_TB_ego) -> Turbine Thermal/3(T_TB_ego1)
  Product/1 -> Turbine Thermal/2(a_ego)
  pedal_toDyno/1 -> Turbine Thermal1/2(pedal_ego)
  Ne_toDyno/1 -> Turbine Thermal1/1(Ne_ego)
  Memory/1 -> Sum/1
  Sum/1 -> Product/2
  Constant/1 -> Product/1
  b_TTB_in_loop/1 -> Switch/2
  Turbine Thermal1/1(T_TB_ego) -> TTB/2, Switch/3, To Workspace8/1, Turbine Thermal1/3(T_TB_ego1)  "TTB_sim"
  T_TB_meas/1 -> TTB/1, Switch/1
  Switch/1 -> TTB/3, TTB_feedback/1

== system VehicleModel/E2C_model/PT1_1 ==
  T_constant : Inport
  in : Inport  Port=2
  T_sample : Inport  Port=3
  map_error_1 : Sum  Inputs=+-  SaturateOnIntegerOverflow=on  InputSameDT=on  OutDataTypeStr=Inherit: Same as first input
  map_error_2 : Sum  Inputs=2  SaturateOnIntegerOverflow=on  InputSameDT=on  OutDataTypeStr=Inherit: Same as first input
  product_1 : Product  Inputs=*/  SaturateOnIntegerOverflow=on  InputSameDT=on  OutDataTypeStr=Inherit: Same as first input
  product_2 : Product  Inputs=**  SaturateOnIntegerOverflow=on  InputSameDT=on  OutDataTypeStr=Inherit: Same as first input
  saturation_1 : Saturate  UpperLimit=1  LowerLimit=0
  unit_delay_1 : UnitDelay  SampleTime=-1
  out : Outport
  wires:
  T_constant/1 -> product_1/2
  T_sample/1 -> product_1/1
  in/1 -> map_error_1/1
  map_error_1/1 -> product_2/2
  product_1/1 -> saturation_1/1
  saturation_1/1 -> product_2/1
  unit_delay_1/1 -> map_error_1/2, map_error_2/2
  map_error_2/1 -> out/1, unit_delay_1/1
  product_2/1 -> map_error_2/1

== system VehicleModel/E2C_model/PT1_2 ==
  T_constant : Inport
  in : Inport  Port=2
  T_sample : Inport  Port=3
  map_error_1 : Sum  Inputs=+-  SaturateOnIntegerOverflow=on  InputSameDT=on  OutDataTypeStr=Inherit: Same as first input
  map_error_2 : Sum  Inputs=2  SaturateOnIntegerOverflow=on  InputSameDT=on  OutDataTypeStr=Inherit: Same as first input
  product_1 : Product  Inputs=*/  SaturateOnIntegerOverflow=on  InputSameDT=on  OutDataTypeStr=Inherit: Same as first input
  product_2 : Product  Inputs=**  SaturateOnIntegerOverflow=on  InputSameDT=on  OutDataTypeStr=Inherit: Same as first input
  saturation_1 : Saturate  UpperLimit=1  LowerLimit=0
  unit_delay_1 : UnitDelay  SampleTime=-1
  out : Outport
  wires:
  T_constant/1 -> product_1/2
  T_sample/1 -> product_1/1
  in/1 -> map_error_1/1
  map_error_1/1 -> product_2/2
  product_1/1 -> saturation_1/1
  saturation_1/1 -> product_2/1
  unit_delay_1/1 -> map_error_1/2, map_error_2/2
  map_error_2/1 -> out/1, unit_delay_1/1
  product_2/1 -> map_error_2/1

== system VehicleModel/E2C_model/noequal ==
  In1 : Inport
  Relational Operator : RelationalOperator  Operator=~=  OutDataTypeStr=boolean  RndMeth=Simplest
  Unit Delay : UnitDelay  SampleTime=-1
  Out1 : Outport
  wires:
  Relational Operator/1 -> Out1/1
  Unit Delay/1 -> Relational Operator/2
  In1/1 -> Unit Delay/1, Relational Operator/1

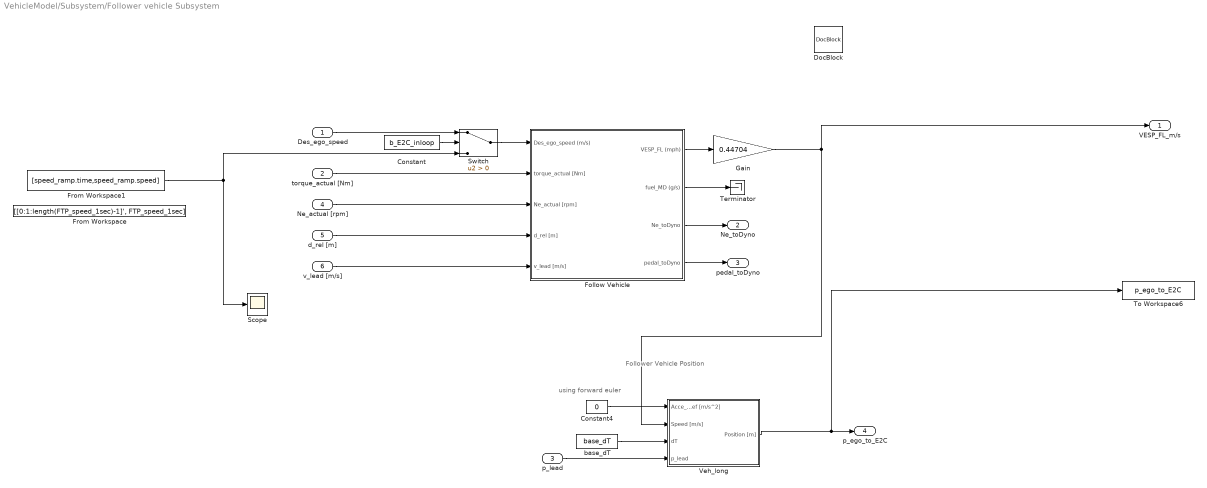
== system VehicleModel/Subsystem/Follower vehicle Subsystem ==
  note: using forward euler
  note: Follower Vehicle Position
  Des_ego_speed : Inport
  torque_actual [Nm] : Inport  Port=2
  p_lead : Inport  Port=3
  Ne_actual [rpm] : Inport  Port=4
  d_rel [m] : Inport  Port=5
  v_lead [m/s] : Inport  Port=6
  Constant : Constant  Value=b_E2C_inloop
  Constant4 : Constant  Value=0
  DocBlock : simulink/Model-Wide Utilities/DocBlock  DocumentType=Text
      content=|
      | Type your documentation here
      |
      | Time
      | 101019T1524         Change Ne profile to be slower by changing Driver_Rsl.
      | 101519T2324         Change torque converter torque_ratio in deceleration to make decel Ne fit better.
      | 102219T1630         Update Gear shift map.
      |                     Use the static Gear shift map depending on (VehV_v,VehV_a)
      |                     Force upshift if engine speed is already >2200 rpm.
      |                     Use filtered V to calculate VehV_a, not the MPC output a_demand.
      | 102519T1650         Change the P and I gain for driver_model to be doubled.
      |                     And then changed back, because with the old P and I gains, fuel matches better with data.
      |                     To solve the Ne and speed tracking problem, saturate Ne integrator by 600 and 3400.
      | 102819T1200         Ddd saturation to match idle fuel, only affect fuel consumption number, do not affect driveline.
      |                     Change GearShifting model to have upshift limits: 1600,1800rpm.
      |                     Second bag when vehicle at move (MD.VESP_mph/2.236>=1.5m/s) fuel consumption:
      |                     data fuel at move is -- 764.1621 [g]
      |                     simulink fuel at move is -- 776.5815 [g], +1.63% error.
      | 102819T2340         Change the "follow vehicle1"-->"gain"0.44 place to before acce_filter.
      |                     Previously "filtered_acce" has unit mph/s...
      |                     Change "follow vehicle1"-->"time constant" from 0.5s to 2s.
      |                     data fuel at move is -- 764.5319 [g]
      |                     simulink fuel at move is -- 771.5589 [g], +1.0% error.
  Follow Vehicle : Subsystem
  From Workspace : FromWorkspace  VariableName=[[0:1:length(FTP_speed_1sec)-1]', FTP_speed_1sec]
  From Workspace1 : FromWorkspace  VariableName=[speed_ramp.time,speed_ramp.speed]
  Gain : Gain  Gain=0.44704
  Scope : Scope
  Switch : Switch  Criteria=u2 > Threshold
  Terminator : Terminator
  To Workspace6 : ToWorkspace  VariableName=p_ego_to_E2C  SaveFormat=Structure With Time  SampleTime=-1
  "Veh_long " : Subsystem
  base_dT : Constant  Value=base_dT
  VESP_FL_m/s : Outport
  Ne_toDyno : Outport  Port=2
  pedal_toDyno : Outport  Port=3
  p_ego_to_E2C : Outport  Port=4
  wires:
  Follow Vehicle/1(VESP_FL (mph)) -> Gain/1
  Follow Vehicle/3(Ne_toDyno) -> Ne_toDyno/1
  Follow Vehicle/4(pedal_toDyno) -> pedal_toDyno/1
  Switch/1 -> Follow Vehicle/1(Des_ego_speed (m/s))
  Des_ego_speed/1 -> Switch/1
  From Workspace1/1 -> Switch/3, Scope/1
  Constant/1 -> Switch/2
  base_dT/1 -> "Veh_long "/3(dT)
  "Veh_long "/1(Position [m]) -> To Workspace6/1, p_ego_to_E2C/1
  Constant4/1 -> "Veh_long "/1(Acce_ref [m/s^2])
  Gain/1 -> VESP_FL_m/s/1, "Veh_long "/2(Speed [m/s])
  torque_actual [Nm]/1 -> Follow Vehicle/2(torque_actual [Nm])
  p_lead/1 -> "Veh_long "/4(p_lead)
  Follow Vehicle/2(fuel_MD (g/s)) -> Terminator/1
  Ne_actual [rpm]/1 -> Follow Vehicle/3(Ne_actual [rpm])
  d_rel [m]/1 -> Follow Vehicle/4(d_rel [m])
  v_lead [m/s]/1 -> Follow Vehicle/5(v_lead [m/s])

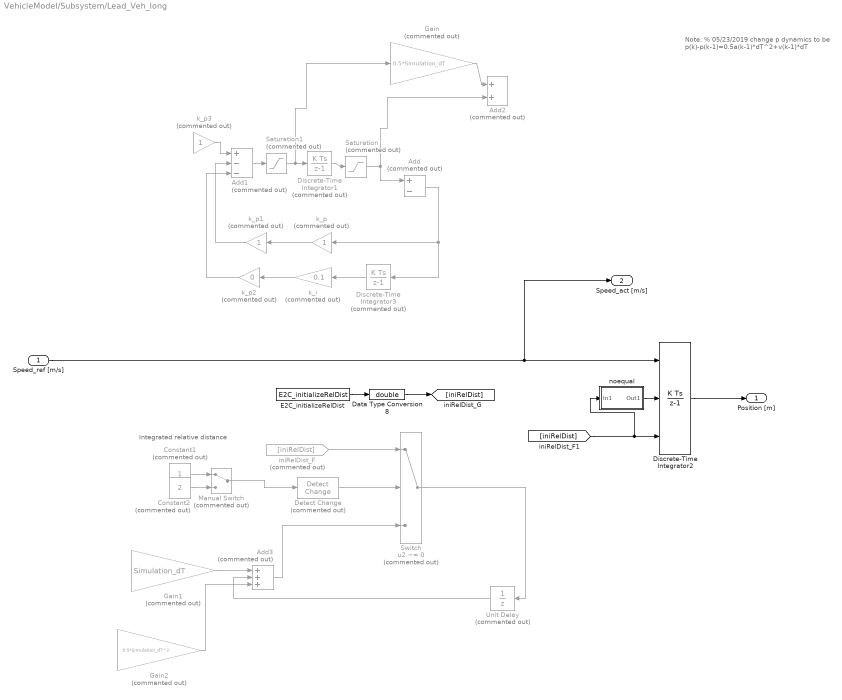
== system VehicleModel/Subsystem/Lead_Veh_long ==
  note: Note:
      | % 05/23/2019
      | change p dynamics to be p(k)-p(k-1)=0.5a(k-1)*dT^2+v(k-1)*dT
  note: Integrated relative distance
  Speed_ref [m/s] : Inport
  Add : Sum  Commented=on  Inputs=+-
  Add1 : Sum  Commented=on  Inputs=+--
  Add2 : Sum  Commented=on
  Add3 : Sum  Commented=on  Inputs=+++
  Constant1 : Constant  Commented=on
  Constant2 : Constant  Commented=on  Value=2
  Data Type Conversion8 : DataTypeConversion  OutDataTypeStr=double
  Detect Change : simulink/Logic and Bit Operations/Detect Change  Commented=on  vinit=0  OutDataTypeStr=boolean
  Discrete-Time Integrator1 : DiscreteIntegrator  Commented=on  InitialCondition=v_lead_ini  InitialConditionSetting=State (most efficient)  SampleTime=-1  ICPrevOutput=DiscIntNeverNeededParam  ICPrevScaledInput=DiscIntNeverNeededParam
  Discrete-Time Integrator2 : DiscreteIntegrator  ExternalReset=rising  InitialConditionSource=external  InitialCondition=p_lead_ini  SampleTime=-1  ICPrevOutput=DiscIntNeverNeededParam  ICPrevScaledInput=DiscIntNeverNeededParam
  Discrete-Time Integrator3 : DiscreteIntegrator  Commented=on  InitialConditionSetting=State (most efficient)  SampleTime=-1  ICPrevOutput=DiscIntNeverNeededParam  ICPrevScaledInput=DiscIntNeverNeededParam
  E2C_initializeRelDist : Constant  Value=E2C_initializeRelDist  OutDataTypeStr=double
  Gain : Gain  Commented=on  Gain=0.5*Simulation_dT
  Gain1 : Gain  Commented=on  Gain=Simulation_dT
  Gain2 : Gain  Commented=on  Gain=0.5*Simulation_dT^2
  Manual Switch : ManualSwitch  Commented=on
  Saturation : Saturate  Commented=on  UpperLimit=30  LowerLimit=0
  Saturation1 : Saturate  Commented=on  UpperLimit=6  LowerLimit=-6
  Switch : Switch  Commented=on  Criteria=u2 ~= 0
  Unit Delay : UnitDelay  Commented=on  SampleTime=-1
  iniRelDist_F : From  Commented=on  GotoTag=iniRelDist
  k_i : Gain  Commented=on  Gain=0.1
  k_p : Gain  Commented=on
  k_p1 : Gain  Commented=on
  k_p2 : Gain  Commented=on  Gain=0
  k_p3 : Gain  Commented=on
  noequal : Subsystem
      mask Display: fprintf('U ~= U/z')
  Position [m] : Outport
  Speed_act [m/s] : Outport  Port=2
  wires:
  Switch/1 -> Unit Delay/1
  Add/1 -> Discrete-Time Integrator3/1, k_p/1
  Discrete-Time Integrator3/1 -> k_i/1
  k_i/1 -> k_p2/1
  k_p/1 -> k_p1/1
  k_p1/1 -> Add1/2
  k_p2/1 -> Add1/3
  Add1/1 -> Saturation1/1
  Discrete-Time Integrator1/1 -> Saturation/1
  k_p3/1 -> Add1/1
  Saturation/1 -> Add2/2, Add/1
  Gain/1 -> Add2/1
  Speed_ref [m/s]/1 -> Speed_act [m/s]/1, Discrete-Time Integrator2/1
  Saturation1/1 -> Discrete-Time Integrator1/1, Gain/1
  iniRelDist_F/1 -> Switch/1
  Detect Change/1 -> Switch/2
  Add3/1 -> Switch/3
  Unit Delay/1 -> Add3/2
  Gain1/1 -> Add3/1
  Gain2/1 -> Add3/3
  Constant1/1 -> Manual Switch/1
  Constant2/1 -> Manual Switch/2
  Manual Switch/1 -> Detect Change/1
  Discrete-Time Integrator2/1 -> Position [m]/1
  [iniRelDist] -> noequal/1(In1), Discrete-Time Integrator2/3
  noequal/1(Out1) -> Discrete-Time Integrator2/2
  E2C_initializeRelDist/1 -> Data Type Conversion8/1
  Data Type Conversion8/1 -> [iniRelDist]

== system VehicleModel/Turbine/Turbine Thermal ==
  v_ego : Inport
  a_ego : Inport  Port=2
  T_TB_ego1 : Inport  Port=3
  Add : Sum  Inputs=+-
  Constant : Constant  Value=T_TB_ego_ini
  Data Type Conversion1 : DataTypeConversion  OutDataTypeStr=double
  Data Type Conversion9 : DataTypeConversion  OutDataTypeStr=double
  Discrete-Time Integrator : DiscreteIntegrator  InitialConditionSource=external  InitialCondition=T_TB_ego_ini  SampleTime=-1  ICPrevOutput=DiscIntNeverNeededParam  ICPrevScaledInput=DiscIntNeverNeededParam
  Divide : Product  Inputs=*/
  E2C_c2_dTB : Constant  Value=E2C_c2_dTB  OutDataTypeStr=double
  E2C_c_dTB : Constant  Value=E2C_c_dTB  OutDataTypeStr=double
  Integrator : Integrator  Commented=on  InitialConditionSource=external  LimitOutput=on  UpperSaturationLimit=3000  LowerSaturationLimit=600
  Product : Product
  Sum : Sum  Inputs=|++
  "Table, Inp.mf_exh" : Lookup_n-D  BreakpointsForDimension1=[0:0.1:30]  BreakpointsForDimension2=[-6:0.1:6]  Table=Inp_mf_exh_par'  InternalRulePriority=Speed  RndMeth=Simplest  InputSameDT=on
  "Table, T_eu" : Lookup_n-D  BreakpointsForDimension1=[0:0.1:30]  BreakpointsForDimension2=[-6:0.1:6]  Table=Inp_t_eu_par'  InternalRulePriority=Speed  RndMeth=Simplest  InputSameDT=on
  T_TB_ego : Outport
  wires:
  "Table, Inp.mf_exh"/1 -> Sum/1
  "Table, T_eu"/1 -> Add/1
  Add/1 -> Product/1
  a_ego/1 -> "Table, Inp.mf_exh"/2, "Table, T_eu"/2
  v_ego/1 -> "Table, Inp.mf_exh"/1, "Table, T_eu"/1
  Product/1 -> Discrete-Time Integrator/1
  Discrete-Time Integrator/1 -> T_TB_ego/1
  T_TB_ego1/1 -> Add/2
  Divide/1 -> Product/2
  E2C_c_dTB/1 -> Data Type Conversion9/1
  Data Type Conversion9/1 -> Divide/2
  Data Type Conversion1/1 -> Sum/2
  Sum/1 -> Divide/1
  E2C_c2_dTB/1 -> Data Type Conversion1/1
  Constant/1 -> Discrete-Time Integrator/2, Integrator/2

== system VehicleModel/Turbine/Turbine Thermal1 ==
  Ne_ego : Inport
  pedal_ego : Inport  Port=2
  T_TB_ego1 : Inport  Port=3
  Add : Sum  Inputs=+-
  Constant : Constant  Value=T_TB_ego_ini
  Data Type Conversion1 : DataTypeConversion  OutDataTypeStr=double
  Data Type Conversion9 : DataTypeConversion  OutDataTypeStr=double
  Discrete-Time Integrator : DiscreteIntegrator  InitialConditionSource=external  InitialCondition=T_TB_ego_ini  SampleTime=-1  ICPrevOutput=DiscIntNeverNeededParam  ICPrevScaledInput=DiscIntNeverNeededParam
  Divide : Product  Inputs=*/
  E2C_c2_dTB : Constant  Value=E2C_c2_dTB  OutDataTypeStr=double
  E2C_c_dTB : Constant  Value=E2C_c_dTB  OutDataTypeStr=double
  Gain1 : Gain  Gain=100  SaturateOnIntegerOverflow=on  OutDataTypeStr=Inherit: Same as input  ParamDataTypeStr=Inherit: Same as input
  Product : Product
  Sum : Sum  Inputs=|++
  TeuMD : Lookup_n-D  BreakpointsForDimension1=PedalMapMD.X  BreakpointsForDimension2=PedalMapMD.Y  Table=PedalMapMD.Teu'  ExtrapMethod=Clip  UseLastTableValue=on  InternalRulePriority=Speed  RndMeth=Simplest  InputSameDT=on
  mexhMD : Lookup_n-D  BreakpointsForDimension1=PedalMapMD.X  BreakpointsForDimension2=PedalMapMD.Y  Table=PedalMapMD.mexh'  ExtrapMethod=Clip  UseLastTableValue=on  InternalRulePriority=Speed  RndMeth=Simplest  InputSameDT=on
  T_TB_ego : Outport
  wires:
  mexhMD/1 -> Sum/1
  TeuMD/1 -> Add/1
  Add/1 -> Product/1
  pedal_ego/1 -> Gain1/1
  Ne_ego/1 -> mexhMD/2, TeuMD/2
  Product/1 -> Discrete-Time Integrator/1
  Discrete-Time Integrator/1 -> T_TB_ego/1
  T_TB_ego1/1 -> Add/2
  Divide/1 -> Product/2
  E2C_c_dTB/1 -> Data Type Conversion9/1
  Data Type Conversion9/1 -> Divide/2
  Data Type Conversion1/1 -> Sum/2
  Sum/1 -> Divide/1
  E2C_c2_dTB/1 -> Data Type Conversion1/1
  Constant/1 -> Discrete-Time Integrator/2
  Gain1/1 -> mexhMD/1, TeuMD/1
